simulink model "Genpath_Simulink"  (R2018b)
settings: Solver=VariableStepAuto  StartTime=0.0  StopTime=0.8  FixedStep=0.001  RelTol=1e-3
values from neighbouring files (symbols this model uses):
  a = Jp/r2^4    (= 12.3456790123)    [Genpath_Optimization.m]
  k = kvar(yindex)    [Genpath_Optimization.m]
  Kt = 0.048    [Genpath_Optimization.m]
  L = Lvar(yindex)    [Genpath_Optimization.m]
  m = mvar(yindex)    [Genpath_Optimization.m]
  r1 = r1var(yindex)    [Genpath_Optimization.m]
  r2 = r2var(yindex)    [Genpath_Optimization.m]
  Rg = 50    [Genpath_Optimization.m]
  Rl = Rlvar(yindex)    [Genpath_Optimization.m]
undefined symbols (not defined in the file or in its folder): sigbuilder_block
settings Model: Creator=GP  LastModifiedBy=thiti
settings SFSimCC: SimUseLocalCustomCode=off
settings RTWCC: RTWUseLocalCustomCode=off

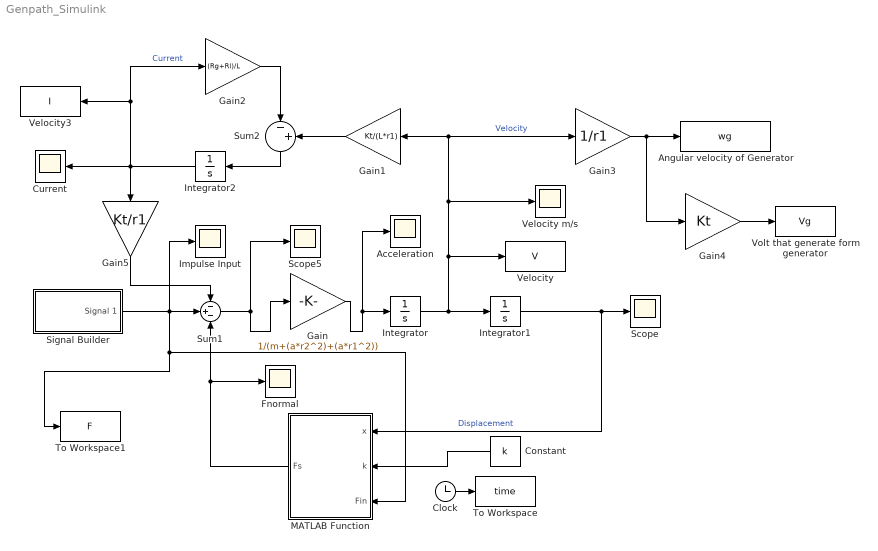
== system Genpath_Simulink ==
  Acceleration : Scope
  Angular velocity of Generator : ToWorkspace  VariableName=wg  SampleTime=-1
  Clock : Clock
  Constant : Constant  Value=k
  Current : Scope
  Fnormal : Scope
  Gain : Gain  Gain=1/(m+(a*r2^2)+(a*r1^2))
  Gain1 : Gain  Gain=Kt/(L*r1)
  Gain2 : Gain  Gain=(Rg+Rl)/L
  Gain3 : Gain  Gain=1/r1
  Gain4 : Gain  Gain=Kt
  Gain5 : Gain  Gain=Kt/r1
  Impulse Input : Scope
  Integrator : Integrator
  Integrator1 : Integrator
  Integrator2 : Integrator
  MATLAB Function : MATLAB Function  TreatAsAtomicUnit=on
  Scope : Scope
  Scope5 : Scope
  Signal Builder : Subsystem  Tag=STV Subsys  LoadFcn=sigbuilder_block('load');  StartFcn=sigbuilder_block('start');  StopFcn=sigbuilder_block('stop');  ClipboardFcn=sigbuilder_block('clipboard');  mask(Sigbuilder block){tuvar=[0:10]}
      mask help: Simulink:masks:SigbuilderBlock_MD
      mask init:
      | if ~strcmp(get_param(bdroot(gcbh),'SimulationStatus'),'stopped') tuvar = sigbuilder_block('maskInit'); end
      settings: CopyFcn=sigbuilder_block('copy');  DeleteFcn=sigbuilder_block('delete');  ModelCloseFcn=sigbuilder_block('modelClose');  PreSaveFcn=sigbuilder_block('preSave');  PauseFcn=sigbuilder_block('pause');  ContinueFcn=sigbuilder_block('continue');  NameChangeFcn=sigbuilder_block('namechange');  OpenFcn=sigbuilder_block('open',[404.25 158.25 550.5 321.75 ]);  CloseFcn=sigbuilder_block('close');
      mask Display: plot(0, 0, 100, 100,[2, 2, 32, 32, 2], [68, 8, 8, 68, 68],[32, 2], [38, 38], [32, 19, 2],[53, 60, 44], [32, 17, 17, 2],[16, 16, 31, 31]);txt = getActiveGroup(gcbh);text(2, 100, txt,'verticalAlignment', 'top');
  Sum1 : Sum  Inputs=-+-
  Sum2 : Sum  Inputs=|-+
  To Workspace : ToWorkspace  VariableName=time  SampleTime=-1
  To Workspace1 : ToWorkspace  VariableName=F  SaveFormat=Timeseries  SampleTime=-1
  Velocity : ToWorkspace  VariableName=V  SampleTime=-1
  Velocity m/s : Scope
  Velocity3 : ToWorkspace  VariableName=I  SampleTime=-1
  Volt that generate form generator : ToWorkspace  VariableName=Vg  SampleTime=-1
  wires:
  Integrator/1 -> Gain3/1, Gain1/1, Velocity m/s/1, Velocity/1, Integrator1/1  "Velocity"
  Gain/1 -> Acceleration/1, Integrator/1
  Sum1/1 -> Scope5/1, Gain/1
  Clock/1 -> To Workspace/1
  MATLAB Function/1(Fs) -> Sum1/3, Fnormal/1
  Integrator1/1 -> MATLAB Function/1(x), Scope/1  "Displacement"
  Signal Builder/1(Signal 1) -> Sum1/2, Impulse Input/1, To Workspace1/1, MATLAB Function/3(Fin)
  Gain1/1 -> Sum2/2
  Sum2/1 -> Integrator2/1
  Integrator2/1 -> Gain5/1, Current/1, Velocity3/1, Gain2/1  "Current"
  Gain2/1 -> Sum2/1
  Gain3/1 -> Gain4/1, Angular velocity of Generator/1
  Gain4/1 -> Volt that generate form generator/1
  Constant/1 -> MATLAB Function/2(k)
  Gain5/1 -> Sum1/1

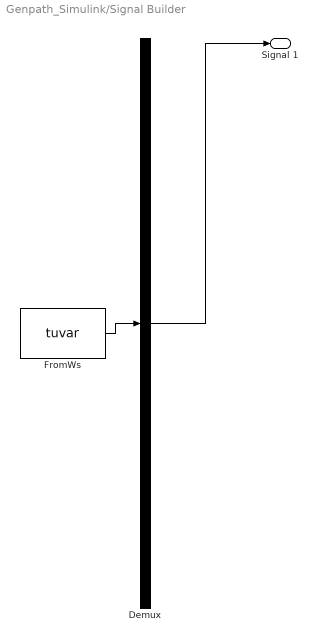
== system Genpath_Simulink/Signal Builder ==
  Demux : Demux  Tag=STV Demux  Outputs=1
  FromWs : FromWorkspace  Tag=STV FromWs  VariableName=tuvar  SampleTime=0
      SigBuilderData=|
      | common.afterFinalStr = 'Extrapolate'
      | common.sampleTime = 0
      | dataSet.timeRange = [0 10]
      | dataSet.name = 'Group 1'
      | sbobj.Groups.Name = 'Group 1'
      | sbobj.Groups.Signals.Name = 'Signal 1'
      | sbobj.Groups.Signals.XData = [0 0.8 0.8 10]
      | sbobj.Groups.Signals.YData = [5 600 0 0]
  Signal 1 : Outport  Tag=STV Outport
  wires:
  Demux/1 -> Signal 1/1
  FromWs/1 -> Demux/1

== matlab function Genpath_Simulink/MATLAB Function ==
  data: x input; k input; Fs output; Fin input
function Fs = fcn(x,k,Fin)

if (x<0.02)
    Fs = k*x;
else
    Fs = Fin;
end
